simulink model "lqg_linear"  (R2022a)
settings: Solver=VariableStepAuto  StartTime=0.0  StopTime=5  MaxStep=0.001  RelTol=1e-3
undefined symbols (not defined in the file): A, B, C, D, E_eps, E_f, K, L
settings Model: Creator=USER  LastModifiedBy=Family
settings SolverCC: AlgebraicLoopSolver=TrustRegion
settings DebuggingCC: UnconnectedInputMsg=warning  UnconnectedOutputMsg=warning  UnconnectedLineMsg=warning  SFMachineParentedDataDiag=warning
settings RTWCC: DLArmComputeVersion=19.05

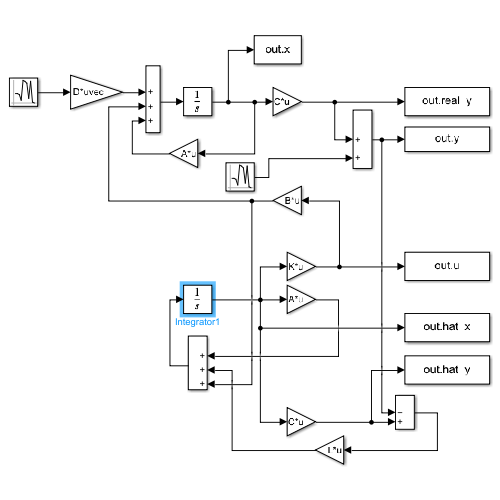
[thumbnail: Simulink's stored preview of the top-level diagram]
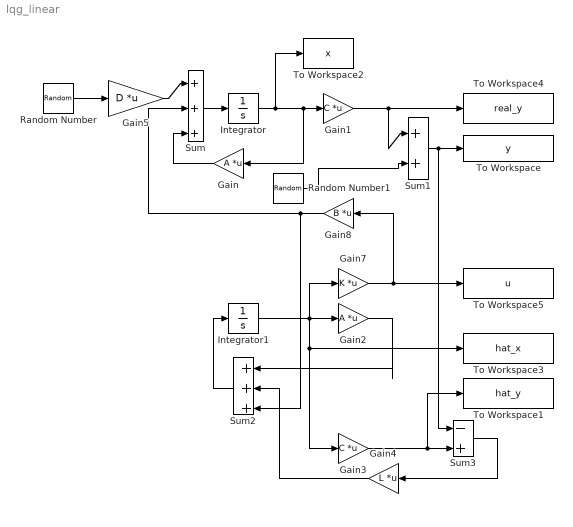
== system lqg_linear ==
  Gain : Gain  Gain=A  Multiplication=Matrix(K*u)
  Gain1 : Gain  Gain=C  Multiplication=Matrix(K*u)
  Gain2 : Gain  Gain=A  Multiplication=Matrix(K*u)
  Gain3 : Gain  Gain=C  Multiplication=Matrix(K*u)
  Gain4 : Gain  Gain=L  Multiplication=Matrix(K*u)
  Gain5 : Gain  Gain=D  Multiplication=Matrix(K*u) (u vector)
  Gain7 : Gain  Gain=K  Multiplication=Matrix(K*u)
  Gain8 : Gain  Gain=B  Multiplication=Matrix(K*u)
  Integrator : Integrator  InitialCondition=[-1;0.1;10;1;5;1]
  Integrator1 : Integrator  InitialCondition=[1;0;1;0;0;2]
  Random Number : RandomNumber  Variance=E_f  Seed=[5 1]  SampleTime=0.1
  Random Number1 : RandomNumber  Variance=E_eps  Seed=1  SampleTime=0.1
  Sum : Sum  Inputs=|+++
  Sum1 : Sum  Inputs=|++
  Sum2 : Sum  Inputs=|+++
  Sum3 : Sum  Inputs=|-+
  To Workspace : ToWorkspace  VariableName=y  SaveFormat=Timeseries  SampleTime=-1
  To Workspace1 : ToWorkspace  VariableName=hat_y  SaveFormat=Timeseries  SampleTime=-1
  To Workspace2 : ToWorkspace  VariableName=x  SaveFormat=Timeseries  SampleTime=-1
  To Workspace3 : ToWorkspace  VariableName=hat_x  SaveFormat=Timeseries  SampleTime=-1
  To Workspace4 : ToWorkspace  VariableName=real_y  SaveFormat=Timeseries  SampleTime=-1
  To Workspace5 : ToWorkspace  VariableName=u  SaveFormat=Timeseries  SampleTime=-1
  wires:
  Gain5/1 -> Sum/1
  Random Number/1 -> Gain5/1
  Sum1/1 -> Sum3/1, To Workspace/1
  Sum2/1 -> Integrator1/1
  Random Number1/1 -> Sum1/2
  Gain4/1 -> Sum2/2
  Integrator/1 -> Gain/1, Gain1/1, To Workspace2/1
  Gain1/1 -> Sum1/1, To Workspace4/1
  Gain2/1 -> Sum2/1
  Sum3/1 -> Gain4/1
  Integrator1/1 -> Gain3/1, To Workspace3/1, Gain2/1, Gain7/1
  Gain3/1 -> To Workspace1/1, Sum3/2
  Sum/1 -> Integrator/1
  Gain8/1 -> Sum/2, Sum2/3
  Gain/1 -> Sum/3
  Gain7/1 -> To Workspace5/1, Gain8/1
